simulink library "SignalProcessingSensorFusionLib"  (R2018b)
settings: Solver=VariableStepAuto  StartTime=0.0  StopTime=10.0  RelTol=1e-3
undefined symbols (not defined in the file): order, Sq_PosBadGradient, Sq_PosIsFrozen, Sq_PosOutOfBounds, threshold
libraries: simulink x15, hdlsllib x3, $bdroot x2
settings Model: Creator=chwit  LastModifiedBy=Patrick
settings SFSimCC: SimUseLocalCustomCode=off
settings RTWCC: RTWUseLocalCustomCode=off

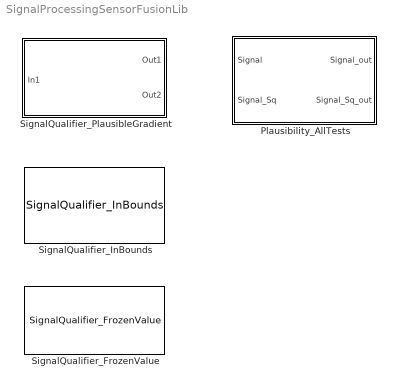
== system SignalProcessingSensorFusionLib ==
  Plausibility_AllTests : Subsystem  mask{alpha=0, checkGradient=on, deviation=0, threshold=0, alpha2=0, increasingPercentage=0, signalBounds=1e-6, stepDelay=3, upperBound=0, lowerBound=0, useAlternativeValue=on, useManualAlternativeValue=off, manualAlternativeValue=0}
      mask prompts: alpha "alpha-value"; checkGradient "Shall the gradient be controlled?"; deviation "gain for accepted deviation"; threshold "Maximal Change per Second"; alpha2 "Inertia of mean (0-1)"; increasingPercentage "percent of the max. changerate add to the allowed deviation [%]"; signalBounds "Signal Bounds"; stepDelay "Step Delay"; upperBound "upper bound"; lowerBound "lower bound"; useAlternativeValue "Shall a alternative value be used if signal is not plausible?"; useManualAlternativeValue "Shall a manually given Value be used? Otherwise signal is held."; manualAlternativeValue "manually given Value"
      mask DialogControl LowPassSettings Prompt: lowpass
      mask DialogControl BadGradientSettings Prompt: bad gradient
      mask DialogControl increasingPercentage Tooltip: How many percent of the max. Change per Second the allowed deviation rises
      mask DialogControl Container8 Prompt: frozen value
      mask DialogControl signalBounds Tooltip: (in which bounds consecutive singals can differ to be detected as frozen )
      mask DialogControl stepDelay Tooltip: how many steps the singal must be within the bounds, so that the signal is detected as frozen
      mask DialogControl Bounds Prompt: bounds
      mask DialogControl AlternativeValue Prompt: alternative Value
      mask DialogControl Container12 Prompt: Use manually given Value
  SignalQualifier_FrozenValue : $bdroot/Plausibility_AllTests/SignalQualifier_FrozenValue  SystemSampleTime=-1
  SignalQualifier_InBounds : $bdroot/Plausibility_AllTests/SignalQualifier_InBounds  SystemSampleTime=-1
  SignalQualifier_PlausibleGradient : Subsystem  mask{timedelay=200, Threshold=100}
      mask prompts: timedelay "Input time delay [ms]"; Threshold "Maximal Gradient per Time Step"

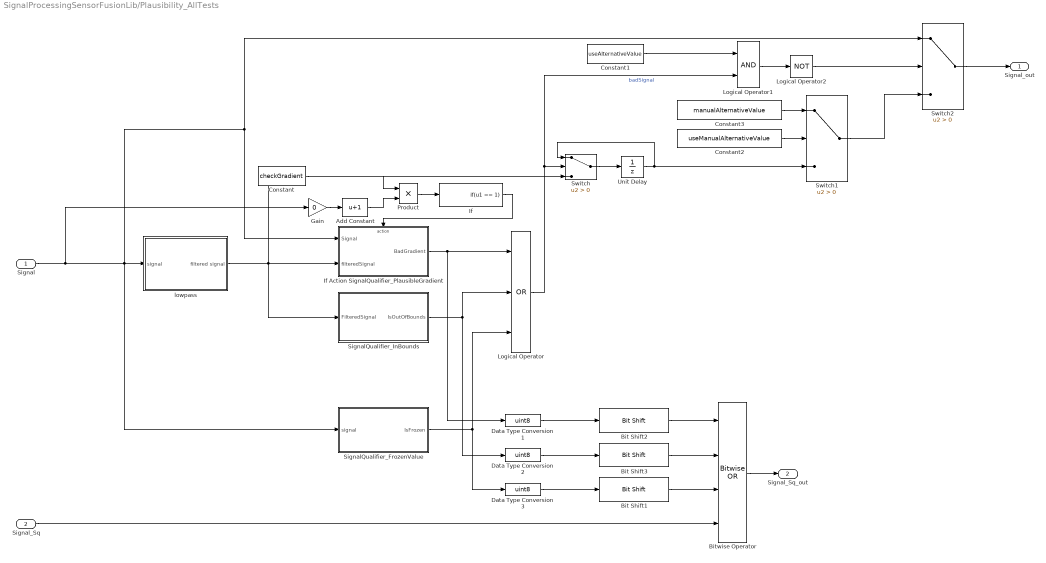
== system SignalProcessingSensorFusionLib/Plausibility_AllTests ==
  Signal : Inport
  Signal_Sq : Inport  Port=2
  Add Constant : Bias  Bias=1
  Bit Shift1 : hdlsllib/Logic and Bit Operations/Bit Shift  mode=Shift Left Logical  N=Sq_PosIsFrozen
      settings: SourceProductName=HDL Coder  SourceProductBaseCode=HD
  Bit Shift2 : hdlsllib/Logic and Bit Operations/Bit Shift  mode=Shift Left Logical  N=Sq_PosBadGradient
      settings: SourceProductName=HDL Coder  SourceProductBaseCode=HD
  Bit Shift3 : hdlsllib/Logic and Bit Operations/Bit Shift  mode=Shift Left Logical  N=Sq_PosOutOfBounds
      settings: SourceProductName=HDL Coder  SourceProductBaseCode=HD
  Bitwise Operator : simulink/Logic and Bit Operations/Bitwise Operator  logicop=OR  UseBitMask=off  NumInputPorts=4  BitMask=bin2dec('11011001')  BitMaskRealWorld=Stored Integer
  Constant : Constant  Value=checkGradient
  Constant1 : Constant  Value=useAlternativeValue
  Constant2 : Constant  Value=useManualAlternativeValue
  Constant3 : Constant  Value=manualAlternativeValue
  Data Type Conversion1 : DataTypeConversion  OutDataTypeStr=uint8
  Data Type Conversion2 : DataTypeConversion  OutDataTypeStr=uint8
  Data Type Conversion3 : DataTypeConversion  OutDataTypeStr=uint8
  Gain : Gain  Gain=0
  If : If  IfExpression=u1 == 1  ShowElse=off
  If Action SignalQualifier_PlausibleGradient : Subsystem  TreatAsAtomicUnit=on
  Logical Operator : Logic  Operator=OR  Inputs=3  AllPortsSameDT=off  OutDataTypeStr=boolean
  Logical Operator1 : Logic  AllPortsSameDT=off  OutDataTypeStr=boolean
  Logical Operator2 : Logic  Operator=NOT  Inputs=1  AllPortsSameDT=off  OutDataTypeStr=boolean
  Product : Product
  SignalQualifier_FrozenValue : Subsystem
  SignalQualifier_InBounds : Subsystem
  Switch : Switch  Criteria=u2 > Threshold
  Switch1 : Switch  Criteria=u2 > Threshold
  Switch2 : Switch  Criteria=u2 > Threshold
  Unit Delay : UnitDelay  SampleTime=-1
  lowpass : Subsystem
  Signal_out : Outport
  Signal_Sq_out : Outport  Port=2
  wires:
  Signal/1 -> Gain/1, SignalQualifier_FrozenValue/1(signal), Switch2/1, If Action SignalQualifier_PlausibleGradient/1(Signal), lowpass/1(signal)
  lowpass/1(filtered signal) -> Switch/3, If Action SignalQualifier_PlausibleGradient/2(filteredSignal), SignalQualifier_InBounds/1(FilteredSignal)
  Bit Shift1/1 -> Bitwise Operator/3
  Bit Shift3/1 -> Bitwise Operator/2
  Signal_Sq/1 -> Bitwise Operator/4
  SignalQualifier_InBounds/1(IsOutOfBounds) -> Data Type Conversion2/1, Logical Operator/2
  SignalQualifier_FrozenValue/1(IsFrozen) -> Logical Operator/3, Data Type Conversion3/1
  If Action SignalQualifier_PlausibleGradient/1(BadGradient) -> Data Type Conversion1/1, Logical Operator/1
  Bitwise Operator/1 -> Signal_Sq_out/1
  Bit Shift2/1 -> Bitwise Operator/1
  Data Type Conversion1/1 -> Bit Shift2/1
  Data Type Conversion2/1 -> Bit Shift3/1
  Data Type Conversion3/1 -> Bit Shift1/1
  Logical Operator/1 -> Switch/2, Logical Operator1/2  "badSignal"
  Constant1/1 -> Logical Operator1/1
  Switch/1 -> Unit Delay/1
  Unit Delay/1 -> Switch1/3, Switch/1
  Constant2/1 -> Switch1/2
  Constant3/1 -> Switch1/1
  Switch2/1 -> Signal_out/1
  Logical Operator1/1 -> Logical Operator2/1
  Logical Operator2/1 -> Switch2/2
  Switch1/1 -> Switch2/3
  If/1 -> If Action SignalQualifier_PlausibleGradient/Action
  Gain/1 -> Add Constant/1
  Add Constant/1 -> Product/2
  Constant/1 -> Product/1
  Product/1 -> If/1

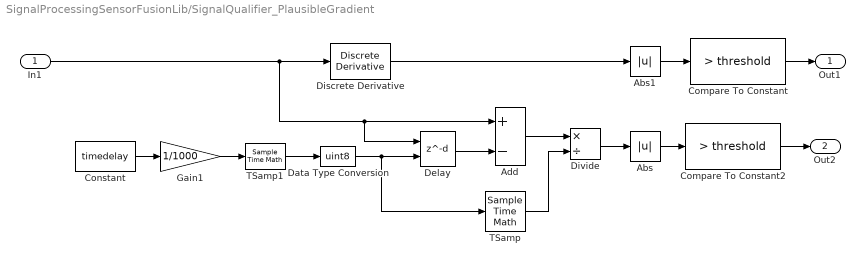
== system SignalProcessingSensorFusionLib/SignalQualifier_PlausibleGradient ==
  In1 : Inport
  Abs : Abs
  Abs1 : Abs
  Add : Sum  Inputs=+-
  Compare To Constant : simulink/Logic and Bit Operations/Compare To Constant  relop=>  const=threshold  OutDataTypeStr=boolean
  Compare To Constant2 : simulink/Logic and Bit Operations/Compare To Constant  relop=>  const=threshold  OutDataTypeStr=boolean
  Constant : Constant  Value=timedelay
  Data Type Conversion : DataTypeConversion  OutDataTypeStr=uint8
  Delay : Delay  DelayLengthSource=Input port  DelayLength=order
      settings: InputPortMap=u0,p1
  Discrete Derivative : simulink/Discrete/Discrete Derivative  gainval=1.0  ICPrevScaledInput=0.0  OutMin=[]  OutMax=[]  OutDataType=fixdt(1, 16)  OutScaling=2^-10  DoSatur=off
  Divide : Product  Inputs=*/
  Gain1 : Gain  Gain=1/1000
  TSamp : SampleTimeMath  DisableCoverage=on  TsampMathOp=*  weightValue=1  TsampMathImp=Offline Scaling Adjustment
  TSamp1 : SampleTimeMath  DisableCoverage=on  TsampMathOp=/  weightValue=1  TsampMathImp=Offline Scaling Adjustment
  Out1 : Outport
  Out2 : Outport  Port=2
  wires:
  In1/1 -> Delay/1, Add/1, Discrete Derivative/1
  Discrete Derivative/1 -> Abs1/1
  Compare To Constant/1 -> Out1/1
  Delay/1 -> Add/2
  Add/1 -> Divide/1
  Abs/1 -> Compare To Constant2/1
  Compare To Constant2/1 -> Out2/1
  TSamp1/1 -> Data Type Conversion/1
  Gain1/1 -> TSamp1/1
  Constant/1 -> Gain1/1
  Data Type Conversion/1 -> TSamp/1, Delay/2
  TSamp/1 -> Divide/2
  Divide/1 -> Abs/1
  Abs1/1 -> Compare To Constant/1

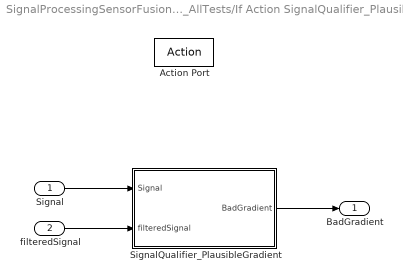
== system SignalProcessingSensorFusionLib/Plausibility_AllTests/If Action SignalQualifier_PlausibleGradient ==
  Signal : Inport
  filteredSignal : Inport  Port=2
  Action Port : ActionPort  ActionType=then
  SignalQualifier_PlausibleGradient : Subsystem
  BadGradient : Outport
  wires:
  Signal/1 -> SignalQualifier_PlausibleGradient/1(Signal)
  filteredSignal/1 -> SignalQualifier_PlausibleGradient/2(filteredSignal)
  SignalQualifier_PlausibleGradient/1(BadGradient) -> BadGradient/1

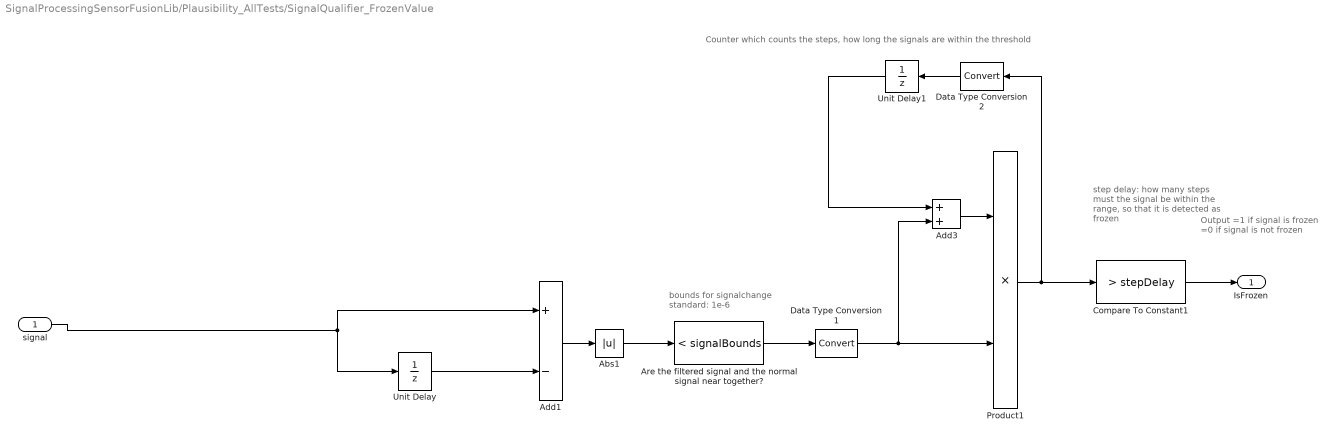
== system SignalProcessingSensorFusionLib/Plausibility_AllTests/SignalQualifier_FrozenValue ==
  note: Output
      | =1 if signal is frozen
      | =0 if signal is not frozen
  note: Counter which counts the steps, how long the signals are within the threshold
  note: bounds for signalchange
      | standard: 1e-6
  note: step delay:
      | how many steps must
      | the signal be within the
      | range, so that it is
      | detected as frozen
  signal : Inport
  Abs1 : Abs
  Add1 : Sum  Inputs=+-
  Add3 : Sum
  Are the filtered signal and the normal signal near together? : simulink/Logic and Bit Operations/Compare To Constant  relop=<  const=signalBounds  OutDataTypeStr=boolean
  Compare To Constant1 : simulink/Logic and Bit Operations/Compare To Constant  relop=>  const=stepDelay  OutDataTypeStr=boolean
  Data Type Conversion1 : DataTypeConversion
  Data Type Conversion2 : DataTypeConversion
  Product1 : Product
  Unit Delay : UnitDelay  SampleTime=-1
  Unit Delay1 : UnitDelay  SampleTime=-1
  IsFrozen : Outport
  wires:
  Add3/1 -> Product1/1
  Data Type Conversion2/1 -> Unit Delay1/1
  Data Type Conversion1/1 -> Product1/2, Add3/2
  Are the filtered signal and the normal signal near together?/1 -> Data Type Conversion1/1
  Unit Delay/1 -> Add1/2
  Add1/1 -> Abs1/1
  Abs1/1 -> Are the filtered signal and the normal signal near together?/1
  Compare To Constant1/1 -> IsFrozen/1
  Unit Delay1/1 -> Add3/1
  Product1/1 -> Compare To Constant1/1, Data Type Conversion2/1
  signal/1 -> Unit Delay/1, Add1/1

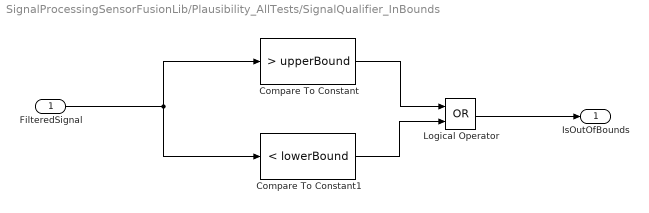
== system SignalProcessingSensorFusionLib/Plausibility_AllTests/SignalQualifier_InBounds ==
  FilteredSignal : Inport
  Compare To Constant : simulink/Logic and Bit Operations/Compare To Constant  relop=>  const=upperBound  OutDataTypeStr=boolean
  Compare To Constant1 : simulink/Logic and Bit Operations/Compare To Constant  relop=<  const=lowerBound  OutDataTypeStr=boolean
  Logical Operator : Logic  Operator=OR  AllPortsSameDT=off  OutDataTypeStr=boolean
  IsOutOfBounds : Outport
  wires:
  Logical Operator/1 -> IsOutOfBounds/1
  Compare To Constant1/1 -> Logical Operator/2
  Compare To Constant/1 -> Logical Operator/1
  FilteredSignal/1 -> Compare To Constant/1, Compare To Constant1/1

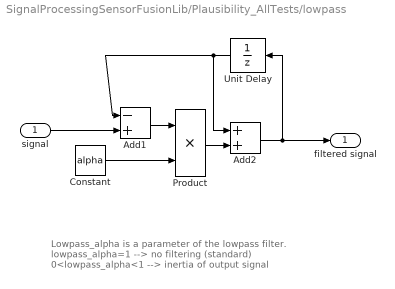
== system SignalProcessingSensorFusionLib/Plausibility_AllTests/lowpass ==
  note: Lowpass_alpha is a parameter of the lowpass filter.
      | lowpass_alpha=1  --> no filtering (standard)
      | 0<lowpass_alpha<1   --> inertia of output signal
  signal : Inport
  Add1 : Sum  Inputs=-+
  Add2 : Sum
  Constant : Constant  Value=alpha
  Product : Product
  Unit Delay : UnitDelay  SampleTime=-1
  filtered signal : Outport
  wires:
  Product/1 -> Add2/2
  Constant/1 -> Product/2
  Unit Delay/1 -> Add2/1, Add1/1
  Add2/1 -> Unit Delay/1, filtered signal/1
  Add1/1 -> Product/1
  signal/1 -> Add1/2

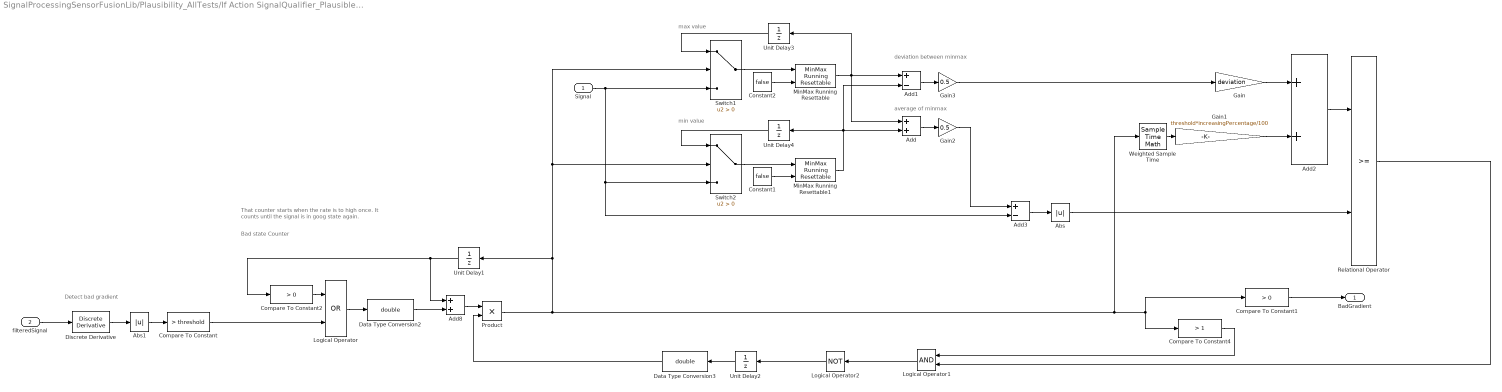
== system SignalProcessingSensorFusionLib/Plausibility_AllTests/If Action SignalQualifier_PlausibleGradient/SignalQualifier_PlausibleGradient ==
  note: deviation between minmax
  note: average of minmax
  note: min value
  note: max value
  note: Bad state Counter
  note: That counter starts when the rate is to high once.
      | It counts until the signal is in goog state again.
  note: Detect bad gradient
  Signal : Inport
  filteredSignal : Inport  Port=2
  Abs : Abs
  Abs1 : Abs
  Add : Sum
  Add1 : Sum  Inputs=+-
  Add2 : Sum
  Add3 : Sum  Inputs=+-
  Add8 : Sum  AccumDataTypeStr=double  OutDataTypeStr=double
  Compare To Constant : simulink/Logic and Bit Operations/Compare To Constant  relop=>  const=threshold  OutDataTypeStr=boolean
  Compare To Constant1 : simulink/Logic and Bit Operations/Compare To Constant  relop=>  const=0  OutDataTypeStr=boolean
  Compare To Constant2 : simulink/Logic and Bit Operations/Compare To Constant  relop=>  const=0  OutDataTypeStr=boolean
  Compare To Constant4 : simulink/Logic and Bit Operations/Compare To Constant  relop=>  const=1  OutDataTypeStr=boolean
  Constant1 : Constant  Value=false
  Constant2 : Constant  Value=false
  Data Type Conversion2 : DataTypeConversion  OutDataTypeStr=double
  Data Type Conversion3 : DataTypeConversion  OutDataTypeStr=double
  Discrete Derivative : simulink/Discrete/Discrete Derivative  gainval=1.0  ICPrevScaledInput=0.0  OutMin=[]  OutMax=[]  OutDataType=fixdt(1, 16)  OutScaling=2^-10  DoSatur=off
  Gain : Gain  Gain=deviation
  Gain1 : Gain  Gain=threshold*increasingPercentage/100
  Gain2 : Gain  Gain=0.5
  Gain3 : Gain  Gain=0.5
  Logical Operator : Logic  Operator=OR  AllPortsSameDT=off  OutDataTypeStr=boolean
  Logical Operator1 : Logic  AllPortsSameDT=off  OutDataTypeStr=boolean
  Logical Operator2 : Logic  Operator=NOT  AllPortsSameDT=off  OutDataTypeStr=boolean
  MinMax Running Resettable : simulink/Math Operations/MinMax Running Resettable  Function=max  vinit=0.0
  MinMax Running Resettable1 : simulink/Math Operations/MinMax Running Resettable  Function=min  vinit=0.0
  Product : Product  OutDataTypeStr=double
  Relational Operator : RelationalOperator  OutDataTypeStr=boolean  RndMeth=Simplest
  Switch1 : Switch  Criteria=u2 > Threshold
  Switch2 : Switch  Criteria=u2 > Threshold
  Unit Delay{1..4} (4 alike) : UnitDelay  SampleTime=-1
  Weighted Sample Time : SampleTimeMath  TsampMathOp=*
  BadGradient : Outport
  wires:
  Weighted Sample Time/1 -> Gain1/1
  Compare To Constant4/1 -> Logical Operator1/1
  Unit Delay2/1 -> Data Type Conversion3/1
  Unit Delay1/1 -> Add8/1, Compare To Constant2/1
  Logical Operator2/1 -> Unit Delay2/1
  Signal/1 -> Switch2/3, Add3/2, Switch1/3
  Data Type Conversion3/1 -> Product/2
  Data Type Conversion2/1 -> Add8/2
  Add8/1 -> Product/1
  Logical Operator1/1 -> Logical Operator2/1
  Relational Operator/1 -> Logical Operator1/2
  Add2/1 -> Relational Operator/1
  Gain1/1 -> Add2/2
  Gain/1 -> Add2/1
  Compare To Constant2/1 -> Logical Operator/1
  Logical Operator/1 -> Data Type Conversion2/1
  Compare To Constant1/1 -> BadGradient/1
  Product/1 -> Switch1/2, Switch2/2, Unit Delay1/1, Weighted Sample Time/1, Compare To Constant4/1, Compare To Constant1/1
  Compare To Constant/1 -> Logical Operator/2
  Abs1/1 -> Compare To Constant/1
  filteredSignal/1 -> Discrete Derivative/1
  Discrete Derivative/1 -> Abs1/1
  Switch1/1 -> MinMax Running Resettable/1
  MinMax Running Resettable/1 -> Add/1, Add1/1, Unit Delay3/1
  Constant2/1 -> MinMax Running Resettable/2
  Constant1/1 -> MinMax Running Resettable1/2
  Switch2/1 -> MinMax Running Resettable1/1
  MinMax Running Resettable1/1 -> Add1/2, Unit Delay4/1, Add/2
  Add/1 -> Gain2/1
  Add1/1 -> Gain3/1
  Gain3/1 -> Gain/1
  Gain2/1 -> Add3/1
  Add3/1 -> Abs/1
  Abs/1 -> Relational Operator/2
  Unit Delay3/1 -> Switch1/1
  Unit Delay4/1 -> Switch2/1
